simulink model "tank_combined_phase4"  (R2025b)
settings: Solver=ode45  StartTime=0.0  StopTime=3600  RelTol=1e-3
libraries: slpidlib x2, simulink x1
settings Model: Creator=maild  LastModifiedBy=maild

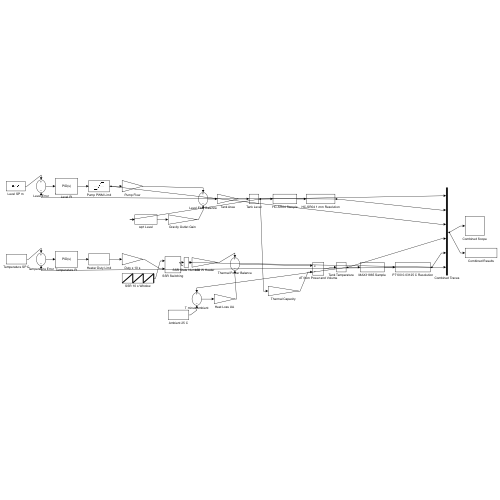
[thumbnail: Simulink's stored preview of the top-level diagram]
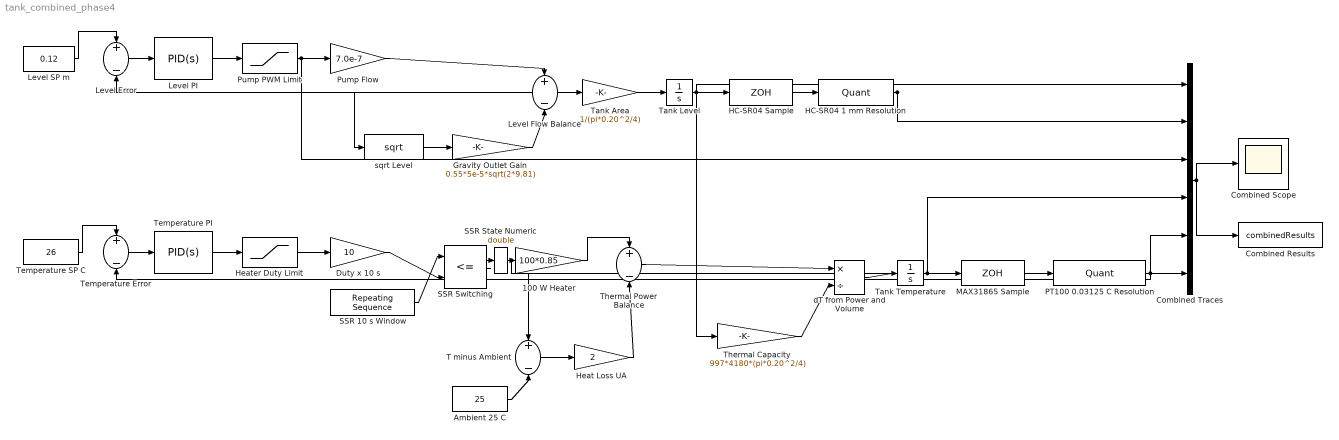
== system tank_combined_phase4 ==
  100 W Heater : Gain  Gain=100*0.85
  Ambient 25 C : Constant  Value=25
  Combined Results : ToWorkspace  VariableName=combinedResults  SaveFormat=Structure With Time  SampleTime=-1
  Combined Scope : Scope
  Combined Traces : Mux  Inputs=6
  Duty x 10 s : Gain  Gain=10
  Gravity Outlet Gain : Gain  Gain=0.55*5e-5*sqrt(2*9.81)
  HC-SR04 1 mm Resolution : Quantizer  QuantizationInterval=0.001
  HC-SR04 Sample : ZeroOrderHold  SampleTime=0.25
  Heat Loss UA : Gain  Gain=2
  Heater Duty Limit : Saturate  UpperLimit=0.10  LowerLimit=0
  Level Error : Sum  Inputs=+-
  Level Flow Balance : Sum  Inputs=+-
  Level PI : slpidlib/PID Controller  Controller=PID  Form=Parallel  TimeDomain=Continuous-time  UseExternalTs=off  SampleTime=-1  IntegratorMethod=Forward Euler  FilterMethod=Forward Euler  ControllerParametersSource=internal  P=1500  I=0.5  UseKiTs=off  D=0  UseExternalDerivativeSource=off  N=100  UseFilter=on  TunerSelectOption=Transfer Function Based (PID Tuner App)  InitialConditionSource=internal  InitialConditionForIntegrator=0  InitialConditionForFilter=0  DifferentiatorICPrevScaledInput=0  ExternalReset=none  TrackingMode=off  Kt=1  LimitOutput=off  SatLimitsSource=internal  UpperSaturationLimit=inf  LowerSaturationLimit=-inf  LinearizeAsGain=on  AntiWindupMode=none  Kb=1  LimitIntegrator=off  UpperIntegratorSaturationLimit=inf  LowerIntegratorSaturationLimit=-inf  POutMin=[]  POutMax=[]  IOutMin=[]  IOutMax=[]  DOutMin=[]  DOutMax=[]  NOutMin=[]  NOutMax=[]  SumOutMin=[]  SumOutMax=[]  SaturationOutMin=[]  SaturationOutMax=[]  PParamMin=[]  PParamMax=[]  IParamMin=[]  IParamMax=[]  DParamMin=[]  DParamMax=[]  NParamMin=[]  NParamMax=[]  KbParamMin=[]  KbParamMax=[]  KtParamMin=[]  KtParamMax=[]  KbOutMin=[]  KbOutMax=[]  KtOutMin=[]  KtOutMax=[]  IntegratorOutMin=[]  IntegratorOutMax=[]  FilterOutMin=[]  FilterOutMax=[]  SumI1OutMin=[]  SumI1OutMax=[]  SumI2OutMin=[]  SumI2OutMax=[]  SumI3OutMin=[]  SumI3OutMax=[]  SumI4OutMin=[]  SumI4OutMax=[]  SumDOutMin=[]  SumDOutMax=[]  DifferentiatorOutMin=[]  DifferentiatorOutMax=[]  FilterDiffOutCoefMin=[]  FilterDiffOutCoefMax=[]  ReciprocalOutMin=[]  ReciprocalOutMax=[]  SumDenOutMin=[]  SumDenOutMax=[]  SumNumOutMin=[]  SumNumOutMax=[]  DivideOutMin=[]  DivideOutMax=[]  UdiffTsProdOutMin=[]  UdiffTsProdOutMax=[]  NTsProdOutMin=[]  NTsProdOutMax=[]  UintegralTsProdOutMin=[]  UintegralTsProdOutMax=[]  UngainTsProdOutMin=[]  UngainTsProdOutMax=[]  ClampingZeroOutDataTypeStr=Inherit: Inherit via back propagation  ClampingZeroOutMin=[]  ClampingZeroOutMax=[]  FilterDenConstantOutDataTypeStr=Inherit: Inherit via back propagation  FilterDenConstantOutMin=[]  FilterDenConstantOutMax=[]  PCopyOutDataTypeStr=Inherit: Inherit via back propagation  PCopyOutMin=[]  PCopyOutMax=[]  NCopyOutDataTypeStr=Inherit: Inherit via back propagation  NCopyOutMin=[]  NCopyOutMax=[]  IntegratorContinuousStateAttributes=''  IntegratorStateMustResolveToSignalObject=off  IntegratorRTWStateStorageClass=Auto  FilterContinuousStateAttributes=''  FilterStateMustResolveToSignalObject=off  FilterRTWStateStorageClass=Auto  ParallelPVariant=InternalParameters  IdealPVariant=Disabled  IVariant=InternalParameters  DVariant=InternalParameters  IntegratorVariant=Continuous  SatVariant=Disabled  AWVariant=Passthrough  PCopyVariant=Disabled  TRVariant=Disabled  FdbkBlocksVariant=Forward  IdealPFdbkVariant=Disabled  SatFdbkVariant=Disabled  DerivativeFilterVariant=ContFilter  NVariant=InternalParameters  NCopyVariant=Disabled  FilterICVariant=InternalICsFilter  IntegratorICVariant=InternalICs  ExternalResetVariant=Disabled  TRSumVariant=Passthrough  SumFdbkVariant=Disabled  SumVariant=Sum_PID  TsampFilterVariant=InternalTs  TsampNgainVariant=Passthrough  TsampIntegralVariant=Disabled_SignalSpec  ExternalSaturationOutDataTypeStr=Inherit: Same as second input  DerivativeSourceVariant=ErrorSignal  PreIntVariant=InternalPreInt
  Level SP m : Constant  Value=0.12
  MAX31865 Sample : ZeroOrderHold  SampleTime=0.021
  PT100 0.03125 C Resolution : Quantizer  QuantizationInterval=0.03125
  Pump Flow : Gain  Gain=7.0e-7
  Pump PWM Limit : Saturate  UpperLimit=100  LowerLimit=0
  SSR 10 s Window : simulink/Sources/Repeating Sequence  rep_seq_t=[0 9.999 10]  rep_seq_y=[0 9.999 0]
  SSR State Numeric : DataTypeConversion  OutDataTypeStr=double  SaturateOnIntegerOverflow=off  RndMeth=Floor
  SSR Switching : RelationalOperator  Operator=<=  OutDataTypeStr=boolean  RndMeth=Simplest  InputSameDT=off
  T minus Ambient : Sum  Inputs=+-
  Tank Area : Gain  Gain=1/(pi*0.20^2/4)
  Tank Level : Integrator  InitialCondition=0.08
  Tank Temperature : Integrator  InitialCondition=25
  Temperature Error : Sum  Inputs=+-
  Temperature PI : slpidlib/PID Controller  Controller=PID  Form=Parallel  TimeDomain=Continuous-time  UseExternalTs=off  SampleTime=-1  IntegratorMethod=Forward Euler  FilterMethod=Forward Euler  ControllerParametersSource=internal  P=0.08  I=0.001  UseKiTs=off  D=0  UseExternalDerivativeSource=off  N=100  UseFilter=on  TunerSelectOption=Transfer Function Based (PID Tuner App)  InitialConditionSource=internal  InitialConditionForIntegrator=0  InitialConditionForFilter=0  DifferentiatorICPrevScaledInput=0  ExternalReset=none  TrackingMode=off  Kt=1  LimitOutput=off  SatLimitsSource=internal  UpperSaturationLimit=inf  LowerSaturationLimit=-inf  LinearizeAsGain=on  AntiWindupMode=none  Kb=1  LimitIntegrator=off  UpperIntegratorSaturationLimit=inf  LowerIntegratorSaturationLimit=-inf  POutMin=[]  POutMax=[]  IOutMin=[]  IOutMax=[]  DOutMin=[]  DOutMax=[]  NOutMin=[]  NOutMax=[]  SumOutMin=[]  SumOutMax=[]  SaturationOutMin=[]  SaturationOutMax=[]  PParamMin=[]  PParamMax=[]  IParamMin=[]  IParamMax=[]  DParamMin=[]  DParamMax=[]  NParamMin=[]  NParamMax=[]  KbParamMin=[]  KbParamMax=[]  KtParamMin=[]  KtParamMax=[]  KbOutMin=[]  KbOutMax=[]  KtOutMin=[]  KtOutMax=[]  IntegratorOutMin=[]  IntegratorOutMax=[]  FilterOutMin=[]  FilterOutMax=[]  SumI1OutMin=[]  SumI1OutMax=[]  SumI2OutMin=[]  SumI2OutMax=[]  SumI3OutMin=[]  SumI3OutMax=[]  SumI4OutMin=[]  SumI4OutMax=[]  SumDOutMin=[]  SumDOutMax=[]  DifferentiatorOutMin=[]  DifferentiatorOutMax=[]  FilterDiffOutCoefMin=[]  FilterDiffOutCoefMax=[]  ReciprocalOutMin=[]  ReciprocalOutMax=[]  SumDenOutMin=[]  SumDenOutMax=[]  SumNumOutMin=[]  SumNumOutMax=[]  DivideOutMin=[]  DivideOutMax=[]  UdiffTsProdOutMin=[]  UdiffTsProdOutMax=[]  NTsProdOutMin=[]  NTsProdOutMax=[]  UintegralTsProdOutMin=[]  UintegralTsProdOutMax=[]  UngainTsProdOutMin=[]  UngainTsProdOutMax=[]  ClampingZeroOutDataTypeStr=Inherit: Inherit via back propagation  ClampingZeroOutMin=[]  ClampingZeroOutMax=[]  FilterDenConstantOutDataTypeStr=Inherit: Inherit via back propagation  FilterDenConstantOutMin=[]  FilterDenConstantOutMax=[]  PCopyOutDataTypeStr=Inherit: Inherit via back propagation  PCopyOutMin=[]  PCopyOutMax=[]  NCopyOutDataTypeStr=Inherit: Inherit via back propagation  NCopyOutMin=[]  NCopyOutMax=[]  IntegratorContinuousStateAttributes=''  IntegratorStateMustResolveToSignalObject=off  IntegratorRTWStateStorageClass=Auto  FilterContinuousStateAttributes=''  FilterStateMustResolveToSignalObject=off  FilterRTWStateStorageClass=Auto  ParallelPVariant=InternalParameters  IdealPVariant=Disabled  IVariant=InternalParameters  DVariant=InternalParameters  IntegratorVariant=Continuous  SatVariant=Disabled  AWVariant=Passthrough  PCopyVariant=Disabled  TRVariant=Disabled  FdbkBlocksVariant=Forward  IdealPFdbkVariant=Disabled  SatFdbkVariant=Disabled  DerivativeFilterVariant=ContFilter  NVariant=InternalParameters  NCopyVariant=Disabled  FilterICVariant=InternalICsFilter  IntegratorICVariant=InternalICs  ExternalResetVariant=Disabled  TRSumVariant=Passthrough  SumFdbkVariant=Disabled  SumVariant=Sum_PID  TsampFilterVariant=InternalTs  TsampNgainVariant=Passthrough  TsampIntegralVariant=Disabled_SignalSpec  ExternalSaturationOutDataTypeStr=Inherit: Same as second input  DerivativeSourceVariant=ErrorSignal  PreIntVariant=InternalPreInt
  Temperature SP C : Constant  Value=26
  Thermal Capacity : Gain  Gain=997*4180*(pi*0.20^2/4)
  Thermal Power Balance : Sum  Inputs=+-
  dT from Power and Volume : Product  Inputs=*/
  sqrt Level : Math  Operator=sqrt
  wires:
  Level SP m/1 -> Level Error/1
  Level Error/1 -> Level PI/1
  Level PI/1 -> Pump PWM Limit/1
  Pump PWM Limit/1 -> Pump Flow/1, Combined Traces/3
  Pump Flow/1 -> Level Flow Balance/1
  Level Flow Balance/1 -> Tank Area/1
  Tank Area/1 -> Tank Level/1
  Tank Level/1 -> HC-SR04 Sample/1, sqrt Level/1, Thermal Capacity/1, Combined Traces/1
  HC-SR04 Sample/1 -> HC-SR04 1 mm Resolution/1
  HC-SR04 1 mm Resolution/1 -> Level Error/2, Combined Traces/2
  sqrt Level/1 -> Gravity Outlet Gain/1
  Gravity Outlet Gain/1 -> Level Flow Balance/2
  Temperature SP C/1 -> Temperature Error/1
  Temperature Error/1 -> Temperature PI/1
  Temperature PI/1 -> Heater Duty Limit/1
  Heater Duty Limit/1 -> Duty x 10 s/1
  SSR 10 s Window/1 -> SSR Switching/1
  Duty x 10 s/1 -> SSR Switching/2
  SSR Switching/1 -> SSR State Numeric/1
  SSR State Numeric/1 -> 100 W Heater/1, Combined Traces/6
  100 W Heater/1 -> Thermal Power Balance/1
  Tank Temperature/1 -> T minus Ambient/1, MAX31865 Sample/1, Combined Traces/4
  Ambient 25 C/1 -> T minus Ambient/2
  T minus Ambient/1 -> Heat Loss UA/1
  Heat Loss UA/1 -> Thermal Power Balance/2
  Thermal Power Balance/1 -> dT from Power and Volume/1
  Thermal Capacity/1 -> dT from Power and Volume/2
  dT from Power and Volume/1 -> Tank Temperature/1
  MAX31865 Sample/1 -> PT100 0.03125 C Resolution/1
  PT100 0.03125 C Resolution/1 -> Temperature Error/2, Combined Traces/5
  Combined Traces/1 -> Combined Scope/1, Combined Results/1
